simulink model "Arcega_HS_SIMULINK_No7"  (R2023b)
settings: Solver=VariableStepAuto  StartTime=0.0  StopTime=20.0  RelTol=1e-3
settings Model: Creator=HANNAH SUZETTE  LastModifiedBy=HANNAH SUZETTE

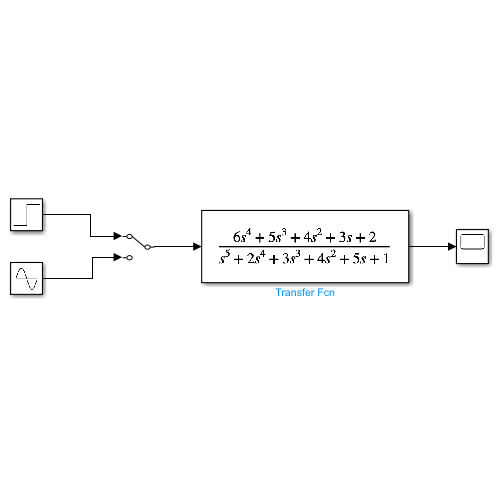
[thumbnail: Simulink's stored preview of the top-level diagram]
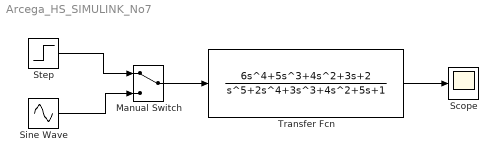
== system Arcega_HS_SIMULINK_No7 ==
  Manual Switch : ManualSwitch
  Scope : Scope
  Sine Wave : Sin  SampleTime=0
  Step : Step  Time=0  SampleTime=0
  Transfer Fcn : TransferFcn  Numerator=[6 5 4 3 2]  Denominator=[1 2 3 4 5 1]
  wires:
  Step/1 -> Manual Switch/1
  Transfer Fcn/1 -> Scope/1
  Sine Wave/1 -> Manual Switch/2
  Manual Switch/1 -> Transfer Fcn/1
